simulink model "Modelo_PO"  (R2023b)
settings: Solver=ode23tb  StartTime=0.0  StopTime=60  RelTol=1e-4
values from neighbouring files (symbols this model uses):
  selector = i    [AA_Simulacion.m]
undefined symbols (not defined in the file or in its folder): sigbuilder_block
libraries: simulink x5, spsSeriesRLCBranchLib x4, spsDiodeLib x2, spsCurrentMeasurementLib x1, spsIGBTLib x1, spsPWMGeneratorDCDCLib x1, spsPVArrayLib x1, spsVoltageMeasurementLib x1, spspowerguiLib x1
settings Model: Creator=Guillermo  LastModifiedBy=Guillermo
settings DebuggingCC: MaskedZcDiagnostic=none  IgnoredZcDiagnostic=none  UnconnectedInputMsg=warning  UnconnectedOutputMsg=warning  UnconnectedLineMsg=warning
settings ModelReferenceCC: EnableRefExpFcnMdlSchedulingChecks=on
settings RTWCC: DLArmComputeVersion=19.05

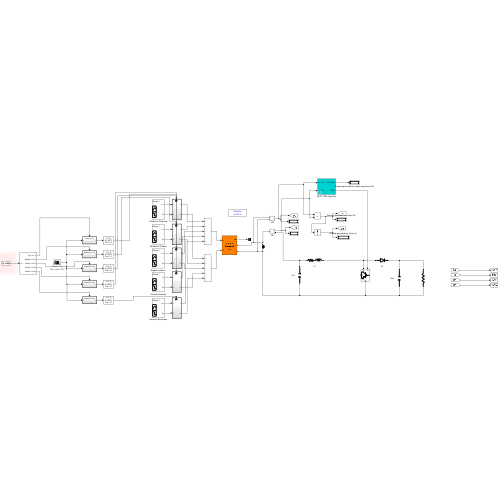
[thumbnail: Simulink's stored preview of the top-level diagram]
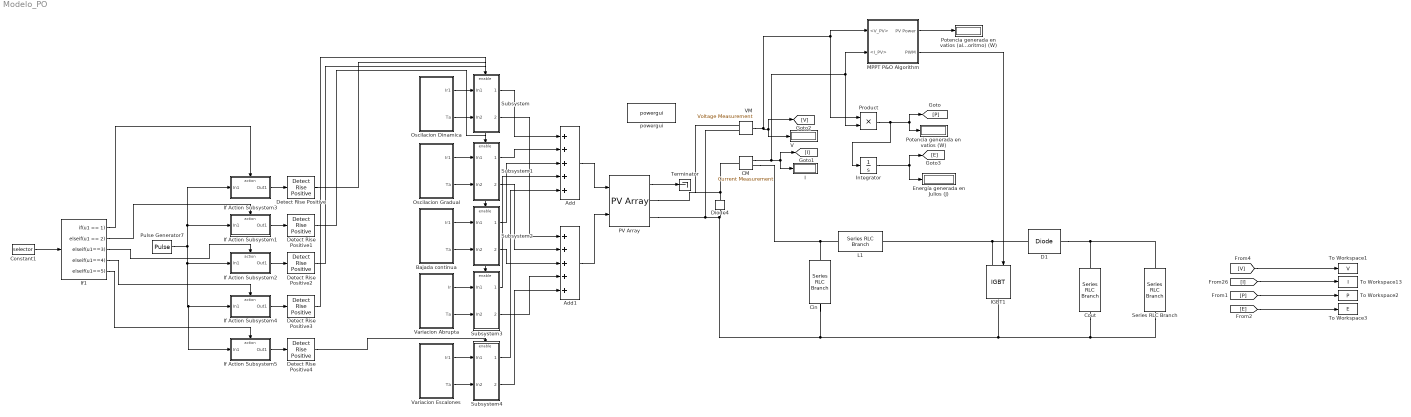
== system Modelo_PO ==
  Add : Sum  Inputs=+++++
  Add1 : Sum  Inputs=+++++
  Bajada continua : Subsystem  Tag=STV Subsys  LoadFcn=sigbuilder_block('load');  StartFcn=sigbuilder_block('start');  StopFcn=sigbuilder_block('stop');  ClipboardFcn=sigbuilder_block('clipboard');  mask(Sigbuilder block){tuvar=[0:10]}
      mask help: Simulink:masks:SigbuilderBlock_MD
      mask init:
      | if ~strcmp(get_param(bdroot(gcbh),'SimulationStatus'),'stopped') tuvar = sigbuilder_block('maskInit'); end
      settings: CopyFcn=sigbuilder_block('copy');  DeleteFcn=sigbuilder_block('delete');  ModelCloseFcn=sigbuilder_block('modelClose');  PreSaveFcn=sigbuilder_block('preSave');  PauseFcn=sigbuilder_block('pause');  ContinueFcn=sigbuilder_block('continue');  NameChangeFcn=sigbuilder_block('namechange');  OpenFcn=sigbuilder_block('open',[6 6 1012.5 506.25 ]);  CloseFcn=sigbuilder_block('close');
      mask Display: plot(0, 0, 100, 100,[2, 2, 32, 32, 2], [68, 8, 8, 68, 68],[32, 2], [38, 38], [32, 19, 2],[53, 60, 44], [32, 17, 17, 2],[16, 16, 31, 31]);txt = getActiveGroup(gcbh);text(2, 100, txt,'verticalAlignment', 'top');
  CM : spsCurrentMeasurementLib/Current Measurement  PhasorSimulation=off  OutputType=Complex  PSBequivalent=0
  Cin : spsSeriesRLCBranchLib/Series RLC Branch  LConnTagsString=__new0  RConnTagsString=__new0  BranchType=C  Resistance=0  Inductance=0  SetiL0=off  InitialCurrent=0  Capacitance=100e-6  Setx0=off  InitialVoltage=0  Measurements=None
  Constant1 : Constant  Value=selector
  Cout : spsSeriesRLCBranchLib/Series RLC Branch  LConnTagsString=__new0  RConnTagsString=__new0  BranchType=C  Resistance=0  Inductance=0  SetiL0=off  InitialCurrent=0  Capacitance=12000e-6  Setx0=off  InitialVoltage=0  Measurements=None
  D1 : spsDiodeLib/Diode  Ron=0.001  Lon=0  Vf=0.8  IC=0  UseSnubber=off  Rs=inf  Cs=250e-9  Measurements=off
  Detect Rise Positive{,1..4} (5 alike) : simulink/Logic and Bit Operations/Detect Rise Positive  vinit=0  OutDataTypeStr=boolean
  Diode4 : spsDiodeLib/Diode  Ron=0.001  Lon=0  Vf=0.7  IC=0  UseSnubber=0  Rs=500  Cs=250e-9  Measurements=off
  "Energía generada en Julios (J) " : Display
  I : Display
  IGBT1 : spsIGBTLib/IGBT  Ron=0.001  Lon=0  Vf=1  Tf=1e-6  Tt=2e-6  IC=0  Rs=1e5  Cs=inf  Measurements=off
  If Action Subsystem1 : Subsystem  TreatAsAtomicUnit=on
  If Action Subsystem2 : Subsystem  TreatAsAtomicUnit=on
  If Action Subsystem3 : Subsystem  TreatAsAtomicUnit=on
  If Action Subsystem4 : Subsystem  TreatAsAtomicUnit=on
  If Action Subsystem5 : Subsystem  TreatAsAtomicUnit=on
  If1 : If  IfExpression=u1 == 1  ElseIfExpressions=u1 == 2, u1==3, u1==4, u1==5  ShowElse=off
  Integrator : Integrator  ZeroCross=off
  L1 : spsSeriesRLCBranchLib/Series RLC Branch  LConnTagsString=__new0  RConnTagsString=__new0  BranchType=RL  Resistance=0  Inductance=0.005  SetiL0=off  InitialCurrent=0  Capacitance=100e-6  Setx0=off  InitialVoltage=0  Measurements=None
  MPPT P&O Algorithm : Subsystem  mask(MPPT Perturb and Observe Algorithm Block){Fsw=1000, StepSize=1e-6}
      mask prompts: Fsw "PWM Switching frequency (Hz):"; StepSize "PWM Duty Cycle (delta) Step Size"
      mask help:
      | MPPT Perturb & Observe Algorithm Block
      | Developed by Rodney Tan (PhD)
      | Version 1.00 Sep 2019
      |
      | This block perform photovoltaic panel Maximum Power Point Tracking based on Perturb & Observe algorithm.
      | This MPPT P&O method is implemented using basic Simulink block only.
      | This MPPT block take in Voltage and Current from photovoltaic panel and output PWM switching signal to drive the DC converter
      mask Help:
      | <b><u>Block Setting</u></b>
      | <b>PWM Switching Frequency (Hz)</b>
      | Specify the PWM switching frequency in Hz.
      | 
      | <b>PWM Duty Cycle Step Size</b>
      | Specify the PWM duty cycle (delta) step size. Default value is 1e-6.
      mask TypeOptions Fsw:
      | PWM Generator
      | (DC-DC)/Fsw
  Oscilacion Dinamica : Subsystem  Tag=STV Subsys  LoadFcn=sigbuilder_block('load');  StartFcn=sigbuilder_block('start');  StopFcn=sigbuilder_block('stop');  ClipboardFcn=sigbuilder_block('clipboard');  mask(Sigbuilder block){tuvar=[0:10]}
      mask help: Simulink:masks:SigbuilderBlock_MD
      mask init:
      | if ~strcmp(get_param(bdroot(gcbh),'SimulationStatus'),'stopped') tuvar = sigbuilder_block('maskInit'); end
      settings: CopyFcn=sigbuilder_block('copy');  DeleteFcn=sigbuilder_block('delete');  ModelCloseFcn=sigbuilder_block('modelClose');  PreSaveFcn=sigbuilder_block('preSave');  PauseFcn=sigbuilder_block('pause');  ContinueFcn=sigbuilder_block('continue');  NameChangeFcn=sigbuilder_block('namechange');  OpenFcn=sigbuilder_block('open',[12.75 -266.25 1012.5 506.25 ]);  CloseFcn=sigbuilder_block('close');
      mask Display: plot(0, 0, 100, 100,[2, 2, 32, 32, 2], [68, 8, 8, 68, 68],[32, 2], [38, 38], [32, 19, 2],[53, 60, 44], [32, 17, 17, 2],[16, 16, 31, 31]);txt = getActiveGroup(gcbh);text(2, 100, txt,'verticalAlignment', 'top');
  Oscilacion Gradual : Subsystem  Tag=STV Subsys  LoadFcn=sigbuilder_block('load');  StartFcn=sigbuilder_block('start');  StopFcn=sigbuilder_block('stop');  ClipboardFcn=sigbuilder_block('clipboard');  mask(Sigbuilder block){tuvar=[0:10]}
      mask help: Simulink:masks:SigbuilderBlock_MD
      mask init:
      | if ~strcmp(get_param(bdroot(gcbh),'SimulationStatus'),'stopped') tuvar = sigbuilder_block('maskInit'); end
      settings: CopyFcn=sigbuilder_block('copy');  DeleteFcn=sigbuilder_block('delete');  ModelCloseFcn=sigbuilder_block('modelClose');  PreSaveFcn=sigbuilder_block('preSave');  PauseFcn=sigbuilder_block('pause');  ContinueFcn=sigbuilder_block('continue');  NameChangeFcn=sigbuilder_block('namechange');  OpenFcn=sigbuilder_block('open',[4.5 30.75 1019.25 481.5 ]);  CloseFcn=sigbuilder_block('close');
      mask Display: plot(0, 0, 100, 100,[2, 2, 32, 32, 2], [68, 8, 8, 68, 68],[32, 2], [38, 38], [32, 19, 2],[53, 60, 44], [32, 17, 17, 2],[16, 16, 31, 31]);txt = getActiveGroup(gcbh);text(2, 100, txt,'verticalAlignment', 'top');
  PV Array : spsPVArrayLib/PV Array  Npar=1  Nser=1  PlotType=array @ 1000 W/m2 & specified temperatures  S_vec="[ 1000  500  100 ]"  Temp_C_vec="[ 45 25  ]"  ModuleName=SunPower SPR-305E-WHT-D  PlotWhenSelected=off  Pm=305.226  Ncell=96  Voc=64.2  Isc=5.96  Vm=54.7  Im=5.58  beta_Voc_pc=-0.2727  alpha_Isc_pc=0.061745  beta_Voc=-0.17507  alpha_Isc=0.00368  IL=5.9657  I0=6.3076e-12  nI=0.94489  Rsh=393.2054  Rs=0.37428  RobustModel=off  RobustCellTemperature=22.6  BAL=on  Tc=1e-3  Tfilter=5e-5
  "Potencia generada en vatios (W) " : Display
  Potencia generada en vatios (algoritmo) (W) : Display
  Product : Product
  Pulse Generator7 : DiscretePulseGenerator  PulseType=Time based  Period=1e-3  PulseWidth=20
      settings: AttributesFormatString=Period: %<period>\nDuty cycle: %<pulsewidth>%
  Series RLC Branch : spsSeriesRLCBranchLib/Series RLC Branch  LConnTagsString=__new0  RConnTagsString=__new0  BranchType=R  Resistance=500  Inductance=1e-3  SetiL0=off  InitialCurrent=0  Capacitance=1e-6  Setx0=off  InitialVoltage=0  Measurements=None
  Subsystem : Subsystem
  Subsystem1 : Subsystem
  Subsystem2 : Subsystem
  Subsystem3 : Subsystem
  Subsystem4 : Subsystem
  Terminator : Terminator
  To Workspace1 : ToWorkspace  VariableName=V  SampleTime=1e-3
  To Workspace13 : ToWorkspace  VariableName=I  SampleTime=1e-3
  To Workspace2 : ToWorkspace  VariableName=P  SampleTime=1e-3
  To Workspace3 : ToWorkspace  VariableName=E  SampleTime=1e-3
  V : Display
  VM : spsVoltageMeasurementLib/Voltage Measurement  PhasorSimulation=off  OutputType=Complex  PSBequivalent=0
  Variacion Abrupta : Subsystem  Tag=STV Subsys  LoadFcn=sigbuilder_block('load');  StartFcn=sigbuilder_block('start');  StopFcn=sigbuilder_block('stop');  ClipboardFcn=sigbuilder_block('clipboard');  mask(Sigbuilder block){tuvar=[0:10]}
      mask help: Simulink:masks:SigbuilderBlock_MD
      mask init:
      | if ~strcmp(get_param(bdroot(gcbh),'SimulationStatus'),'stopped') tuvar = sigbuilder_block('maskInit'); end
      settings: CopyFcn=sigbuilder_block('copy');  DeleteFcn=sigbuilder_block('delete');  ModelCloseFcn=sigbuilder_block('modelClose');  PreSaveFcn=sigbuilder_block('preSave');  PauseFcn=sigbuilder_block('pause');  ContinueFcn=sigbuilder_block('continue');  NameChangeFcn=sigbuilder_block('namechange');  OpenFcn=sigbuilder_block('open',[6 6 1012.5 506.25 ]);  CloseFcn=sigbuilder_block('close');
      mask Display: plot(0, 0, 100, 100,[2, 2, 32, 32, 2], [68, 8, 8, 68, 68],[32, 2], [38, 38], [32, 19, 2],[53, 60, 44], [32, 17, 17, 2],[16, 16, 31, 31]);txt = getActiveGroup(gcbh);text(2, 100, txt,'verticalAlignment', 'top');
  Variacion Escalones : Subsystem  Tag=STV Subsys  LoadFcn=sigbuilder_block('load');  StartFcn=sigbuilder_block('start');  StopFcn=sigbuilder_block('stop');  ClipboardFcn=sigbuilder_block('clipboard');  mask(Sigbuilder block){tuvar=[0:10]}
      mask help: Simulink:masks:SigbuilderBlock_MD
      mask init:
      | if ~strcmp(get_param(bdroot(gcbh),'SimulationStatus'),'stopped') tuvar = sigbuilder_block('maskInit'); end
      settings: CopyFcn=sigbuilder_block('copy');  DeleteFcn=sigbuilder_block('delete');  ModelCloseFcn=sigbuilder_block('modelClose');  PreSaveFcn=sigbuilder_block('preSave');  PauseFcn=sigbuilder_block('pause');  ContinueFcn=sigbuilder_block('continue');  NameChangeFcn=sigbuilder_block('namechange');  OpenFcn=sigbuilder_block('open',[6 6 1012.5 506.25 ]);  CloseFcn=sigbuilder_block('close');
      mask Display: plot(0, 0, 100, 100,[2, 2, 32, 32, 2], [68, 8, 8, 68, 68],[32, 2], [38, 38], [32, 19, 2],[53, 60, 44], [32, 17, 17, 2],[16, 16, 31, 31]);txt = getActiveGroup(gcbh);text(2, 100, txt,'verticalAlignment', 'top');
  powergui : spspowerguiLib/powergui  Priority=1  SimulationMode=Discrete  SampleTime=1e-5  frequency=60  Iterations=50  frequencyindice=0  Pbase=100e6  ErrMax=1e-4  UnitsV=kV  UnitsW=MW  buscounter=0  FunctionMessages=off  echomessages=off  EnableUseOfTLC=off  CurrentSourceSwitches=on  DisableSnubberDevices=on  DisableRonSwitches=off  DisableVfSwitches=off  DisplayEquations=off  AutomaticDiscreteSolvers=off  SolverType=Tustin/Backward Euler (TBE)  Interpol=off  ExternalGateDelay=off  methode=off  Ts=0  x0status=blocks  SPID=off  SwTol=0  HookPort=off  NonlinearTolerance=1e-4  nMaxIteration=100  ContinueOnMaxIteration=off  RestoreLinks=warning  ResistiveCurrentMeasurement=off  Frange=[0:2:500]  Ylog=off  Xlog=on  ShowGrid=off  save=off  variable=ZData  structure=0  ZoomFFT=on  StartTime=0.0  cycles=1  DisplayStyle=1  fundamental=60  FreqAxis=off  MaxFrequency=1000  frequencyindicesteady=1  RmsSteady=1  display=off
  wires:
  [V] -> To Workspace1/1
  VM/1 -> Product/1, MPPT P&O Algorithm/1(<V_PV>), [V], V/1
  CM/1 -> I/1, [I], Product/2, MPPT P&O Algorithm/2(<I_PV>)
  PV Array/1 -> Terminator/1
  [I] -> To Workspace13/1
  Integrator/1 -> [E], "Energía generada en Julios (J) "/1
  [P] -> To Workspace2/1
  [E] -> To Workspace3/1
  MPPT P&O Algorithm/2(PWM) -> IGBT1/1
  MPPT P&O Algorithm/1(PV Power) -> Potencia generada en vatios (algoritmo) (W)/1
  Product/1 -> Integrator/1, "Potencia generada en vatios (W) "/1, [P]
  Subsystem2/1(Out1) -> Add/3
  Subsystem/2(Out2) -> Add1/1
  Subsystem4/1(Out1) -> Add/5
  If Action Subsystem1/1(Out1) -> Detect Rise Positive1/1
  Oscilacion Gradual/1(Ir1) -> Subsystem1/1(In1)
  Oscilacion Dinamica/2(Ta) -> Subsystem/2(In2)
  If Action Subsystem5/1(Out1) -> Detect Rise Positive4/1
  Subsystem/1(Out1) -> Add/1
  Subsystem1/2(Out2) -> Add1/2
  Subsystem2/2(Out2) -> Add1/3
  Subsystem3/2(Out2) -> Add1/4
  Variacion Abrupta/2(Ta) -> Subsystem3/2(In2)
  Oscilacion Dinamica/1(Ir1) -> Subsystem/1(In1)
  If1/1 -> If Action Subsystem3/Action
  Variacion Escalones/2(Ta) -> Subsystem4/2(In2)
  Detect Rise Positive/1 -> Subsystem/Enable
  If1/5 -> If Action Subsystem5/Action
  If Action Subsystem4/1(Out1) -> Detect Rise Positive3/1
  Subsystem4/2(Out2) -> Add1/5
  Variacion Abrupta/1(Ir) -> Subsystem3/1(In1)
  Subsystem3/1(Out1) -> Add/4
  Bajada continua/1(Ir1) -> Subsystem2/1(In1)
  If1/3 -> If Action Subsystem2/Action
  Constant1/1 -> If1/1
  Pulse Generator7/1 -> If Action Subsystem3/1(In1), If Action Subsystem1/1(In1), If Action Subsystem5/1(In1), If Action Subsystem4/1(In1), If Action Subsystem2/1(In1)
  Subsystem1/1(Out1) -> Add/2
  Bajada continua/2(Ta) -> Subsystem2/2(In2)
  If Action Subsystem2/1(Out1) -> Detect Rise Positive2/1
  If1/2 -> If Action Subsystem1/Action
  If1/4 -> If Action Subsystem4/Action
  Variacion Escalones/1(Ir1) -> Subsystem4/1(In1)
  If Action Subsystem3/1(Out1) -> Detect Rise Positive/1
  Oscilacion Gradual/2(Ta) -> Subsystem1/2(In2)
  Add/1 -> PV Array/1
  Add1/1 -> PV Array/2
  Detect Rise Positive1/1 -> Subsystem1/Enable
  Detect Rise Positive2/1 -> Subsystem2/Enable
  Detect Rise Positive3/1 -> Subsystem3/Enable
  Detect Rise Positive4/1 -> Subsystem4/Enable
  connections:
  D1/LConn1 -- IGBT1/LConn1 -- L1/RConn1
  PV Array/RConn2 -- VM/LConn2 -- Cin/RConn1 -- Cout/RConn1 -- Series RLC Branch/RConn1 -- IGBT1/RConn1 -- Diode4/LConn1
  Series RLC Branch/LConn1 -- D1/RConn1 -- Cout/LConn1
  Diode4/RConn1 -- VM/LConn1 -- PV Array/RConn1 -- CM/LConn1
  CM/RConn1 -- Cin/LConn1 -- L1/LConn1

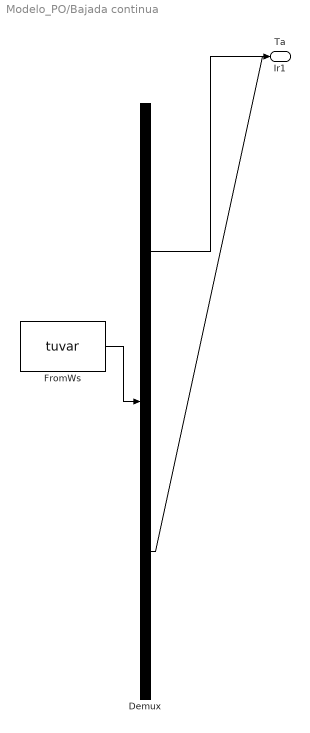
== system Modelo_PO/Bajada continua ==
  Demux : Demux  Tag=STV Demux  Outputs=2
      settings: DisplayOption=none
  FromWs : FromWorkspace  Tag=STV FromWs  VariableName=tuvar
      SigBuilderData=|
      | common.afterFinalStr = 'Extrapolate'
      | common.sampleTime = 0
      | dataSet.timeRange = [0 60]
      | dataSet.name = 'Group 1'
      | sbobj.Groups.Name = 'Group 1'
      | sbobj.Groups.Signals(1).Name = 'Ir1'
      | sbobj.Groups.Signals(1).XData = [0 60]
      | sbobj.Groups.Signals(1).YData = [1000 0]
      | sbobj.Groups.Signals(2).Name = 'Ta'
      | sbobj.Groups.Signals(2).XData = [0 60]
      | sbobj.Groups.Signals(2).YData = [22.6 22.6]
      | sbobj.Groups.TimeRange = [0 60]
  Ir1 : Outport  Tag=STV Outport
  Ta : Outport  Tag=STV Outport  Port=2
  wires:
  FromWs/1 -> Demux/1
  Demux/1 -> Ir1/1
  Demux/2 -> Ta/1

== system Modelo_PO/If Action Subsystem1 ==
  In1 : Inport
  Action Port : ActionPort  InitializeStates=reset  ActionPortLabel=elseif(u1 == 2)
  Out1 : Outport
  wires:
  In1/1 -> Out1/1

== system Modelo_PO/If Action Subsystem2 ==
  In1 : Inport
  Action Port : ActionPort  InitializeStates=reset  ActionPortLabel=elseif( u1==3)
  Out1 : Outport
  wires:
  In1/1 -> Out1/1

== system Modelo_PO/If Action Subsystem3 ==
  In1 : Inport
  Action Port : ActionPort  InitializeStates=reset  ActionPortLabel=if(u1 == 1)
  Out1 : Outport
  wires:
  In1/1 -> Out1/1

== system Modelo_PO/If Action Subsystem4 ==
  In1 : Inport
  Action Port : ActionPort  InitializeStates=reset  ActionPortLabel=elseif( u1==4)
  Out1 : Outport
  wires:
  In1/1 -> Out1/1

== system Modelo_PO/If Action Subsystem5 ==
  In1 : Inport
  Action Port : ActionPort  InitializeStates=reset  ActionPortLabel=elseif( u1==5)
  Out1 : Outport
  wires:
  In1/1 -> Out1/1

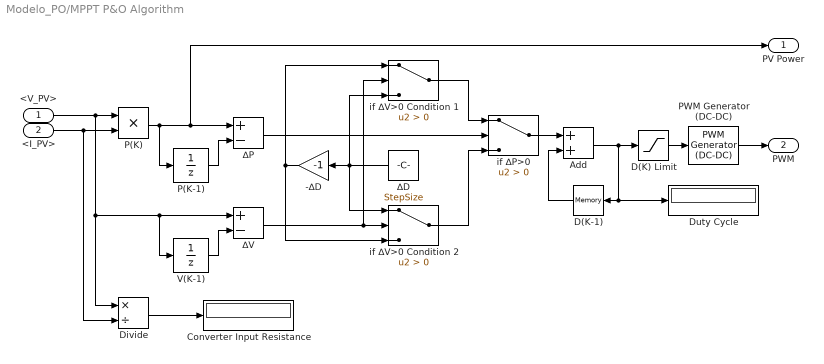
== system Modelo_PO/MPPT P&O Algorithm ==
  <V_PV> : Inport
  <I_PV> : Inport  Port=2
  -∆D : Gain  Gain=-1
  Add : Sum
  Converter Input Resistance : Display
  D(K) Limit : Saturate  UpperLimit=1  LowerLimit=0
  D(K-1) : Memory  InitialCondition=0.5  InheritSampleTime=on
  Divide : Product  Inputs=*/
  Duty Cycle : Display
  P(K) : Product
  P(K-1) : UnitDelay  SampleTime=-1  HasFrameUpgradeWarning=on
  PWM Generator (DC-DC) : spsPWMGeneratorDCDCLib/PWM Generator (DC-DC)  Fsw=Fsw  Ts=0
  V(K-1) : UnitDelay  SampleTime=-1  HasFrameUpgradeWarning=on
  if ∆P>0 : Switch  Criteria=u2 > Threshold  SaturateOnIntegerOverflow=off  InputSameDT=off
  if ∆V>0 Condition 1 : Switch  Criteria=u2 > Threshold  SaturateOnIntegerOverflow=off  InputSameDT=off
  if ∆V>0 Condition 2 : Switch  Criteria=u2 > Threshold  SaturateOnIntegerOverflow=off  InputSameDT=off
  ∆D : Constant  Value=StepSize
  ∆P : Sum  Inputs=+-
  ∆V : Sum  Inputs=+-
  PV Power : Outport  VectorParamsAs1DForOutWhenUnconnected=off
  PWM : Outport  Port=2  VectorParamsAs1DForOutWhenUnconnected=off
  wires:
  P(K)/1 -> ∆P/1, PV Power/1, P(K-1)/1
  <I_PV>/1 -> P(K)/2, Divide/2
  if ∆P>0/1 -> Add/1
  if ∆V>0 Condition 1/1 -> if ∆P>0/1
  ∆P/1 -> if ∆P>0/2
  P(K-1)/1 -> ∆P/2
  V(K-1)/1 -> ∆V/2
  ∆V/1 -> if ∆V>0 Condition 2/2, if ∆V>0 Condition 1/2
  <V_PV>/1 -> Divide/1, ∆V/1, V(K-1)/1, P(K)/1
  Add/1 -> D(K) Limit/1, Duty Cycle/1, D(K-1)/1
  if ∆V>0 Condition 2/1 -> if ∆P>0/3
  D(K-1)/1 -> Add/2
  ∆D/1 -> if ∆V>0 Condition 2/1, -∆D/1, if ∆V>0 Condition 1/3
  -∆D/1 -> if ∆V>0 Condition 2/3, if ∆V>0 Condition 1/1
  PWM Generator (DC-DC)/1 -> PWM/1
  Divide/1 -> Converter Input Resistance/1
  D(K) Limit/1 -> PWM Generator (DC-DC)/1

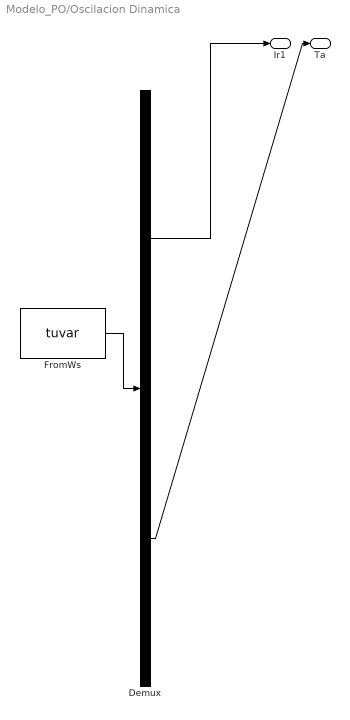
== system Modelo_PO/Oscilacion Dinamica ==
  Demux : Demux  Tag=STV Demux  Outputs=2
      settings: DisplayOption=none
  FromWs : FromWorkspace  Tag=STV FromWs  VariableName=tuvar
      SigBuilderData=|
      | common.afterFinalStr = 'Extrapolate'
      | common.sampleTime = 0
      | dataSet.timeRange = [0 60]
      | dataSet.name = 'Group 1'
      | sbobj.Groups.Name = 'Group 1'
      | sbobj.Groups.Signals(1).Name = 'Ir1'
      | sbobj.Groups.Signals(1).XData = [0 1 1.4 7 7.25 10 10.25 10.5 12 12.25 16 16.25 16.5 16.75 18.95 19.5 20 21.05 24 24.5 25 25.25 25.75 29 32 32.25 34 34.25 34.5 34.75 35 37 37.25 41 41.25 41.5 41.75 42 45 45.25 48 48.25 50 50.25 53.75 54 54.25 57 57.25 60]
      | sbobj.Groups.Signals(1).YData = [910 500 295 295 910 910 295 295 295 910 910 295 910 295 295 910 295 910 910 290 910 295 910 910 910 295 295 910 295 910 295 295 910 910 295 910 295 910 910 295 295 910 910 295 295 910 295 295 790 790]
      | sbobj.Groups.Signals(2).Name = 'Ta'
      | sbobj.Groups.Signals(2).XData = [0 60]
      | sbobj.Groups.Signals(2).YData = [22.6 22.6]
      | sbobj.Groups.TimeRange = [0 60]
  Ir1 : Outport  Tag=STV Outport
  Ta : Outport  Tag=STV Outport  Port=2
  wires:
  FromWs/1 -> Demux/1
  Demux/1 -> Ir1/1
  Demux/2 -> Ta/1

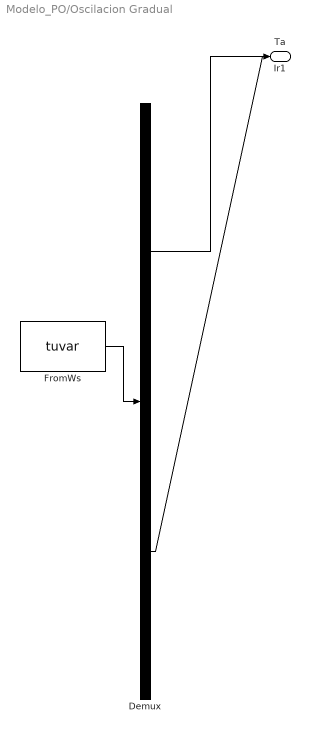
== system Modelo_PO/Oscilacion Gradual ==
  Demux : Demux  Tag=STV Demux  Outputs=2
      settings: DisplayOption=none
  FromWs : FromWorkspace  Tag=STV FromWs  VariableName=tuvar
      SigBuilderData=|
      | common.afterFinalStr = 'Extrapolate'
      | common.sampleTime = 0
      | dataSet.timeRange = [0 60]
      | dataSet.name = 'Group 1'
      | sbobj.Groups.Name = 'Group 1'
      | sbobj.Groups.Signals(1).Name = 'Ir1'
      | sbobj.Groups.Signals(1).XData = [0 1 1.4 7 7.25 16.5 16.75 25.25 25.75 34.75 35 37 37.25 45 45.25 48 48.25 50 50.25 57 57.25 57.25 60]
      | sbobj.Groups.Signals(1).YData = [910 500 295 295 910 910 295 295 910 910 295 295 910 910 295 295 910 910 295 295 775 800 800]
      | sbobj.Groups.Signals(2).Name = 'Ta'
      | sbobj.Groups.Signals(2).XData = [0 60]
      | sbobj.Groups.Signals(2).YData = [22.6 22.6]
      | sbobj.Groups.TimeRange = [0 60]
  Ir1 : Outport  Tag=STV Outport
  Ta : Outport  Tag=STV Outport  Port=2
  wires:
  FromWs/1 -> Demux/1
  Demux/1 -> Ir1/1
  Demux/2 -> Ta/1

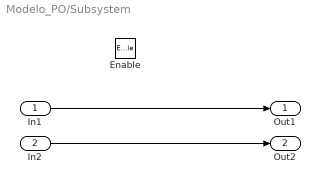
== system Modelo_PO/Subsystem ==
  In1 : Inport
  In2 : Inport  Port=2
  Enable : EnablePort
  Out1 : Outport
  Out2 : Outport  Port=2
  wires:
  In1/1 -> Out1/1
  In2/1 -> Out2/1

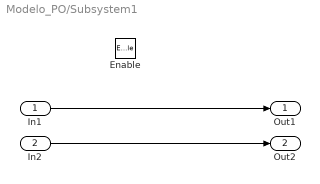
== system Modelo_PO/Subsystem1 ==
  In1 : Inport
  In2 : Inport  Port=2
  Enable : EnablePort
  Out1 : Outport
  Out2 : Outport  Port=2
  wires:
  In1/1 -> Out1/1
  In2/1 -> Out2/1

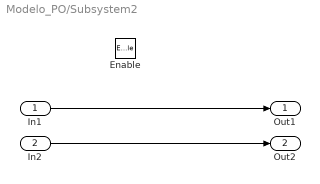
== system Modelo_PO/Subsystem2 ==
  In1 : Inport
  In2 : Inport  Port=2
  Enable : EnablePort
  Out1 : Outport
  Out2 : Outport  Port=2
  wires:
  In1/1 -> Out1/1
  In2/1 -> Out2/1

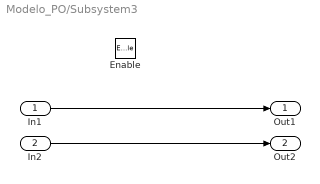
== system Modelo_PO/Subsystem3 ==
  In1 : Inport
  In2 : Inport  Port=2
  Enable : EnablePort
  Out1 : Outport
  Out2 : Outport  Port=2
  wires:
  In1/1 -> Out1/1
  In2/1 -> Out2/1

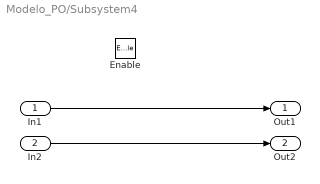
== system Modelo_PO/Subsystem4 ==
  In1 : Inport
  In2 : Inport  Port=2
  Enable : EnablePort
  Out1 : Outport
  Out2 : Outport  Port=2
  wires:
  In1/1 -> Out1/1
  In2/1 -> Out2/1

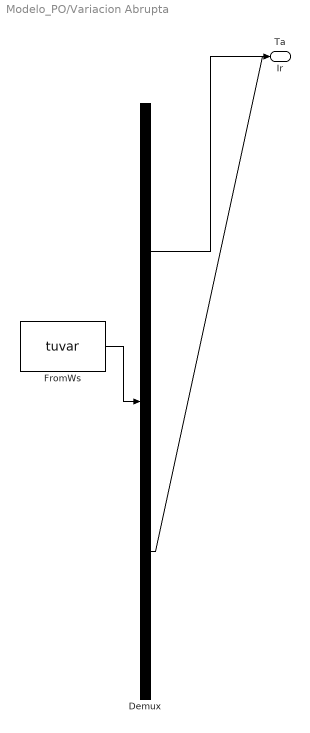
== system Modelo_PO/Variacion Abrupta ==
  Demux : Demux  Tag=STV Demux  Outputs=2
      settings: DisplayOption=none
  FromWs : FromWorkspace  Tag=STV FromWs  VariableName=tuvar
      SigBuilderData=|
      | common.afterFinalStr = 'Extrapolate'
      | common.sampleTime = 0
      | dataSet.timeRange = [0 60]
      | dataSet.name = 'Group 1'
      | sbobj.Groups.Name = 'Group 1'
      | sbobj.Groups.Signals(1).Name = 'Ir'
      | sbobj.Groups.Signals(1).XData = [0 20 20.1 40 40.1 60]
      | sbobj.Groups.Signals(1).YData = [800 800 100 100 600 600]
      | sbobj.Groups.Signals(2).Name = 'Ta'
      | sbobj.Groups.Signals(2).XData = [0 60]
      | sbobj.Groups.Signals(2).YData = [22.6 22.6]
      | sbobj.Groups.TimeRange = [0 60]
  Ir : Outport  Tag=STV Outport
  Ta : Outport  Tag=STV Outport  Port=2
  wires:
  FromWs/1 -> Demux/1
  Demux/1 -> Ir/1
  Demux/2 -> Ta/1

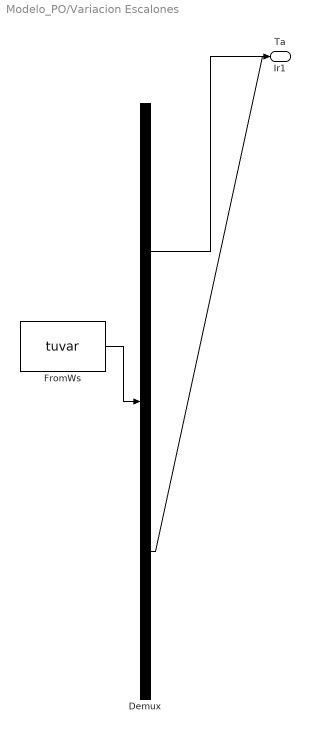
== system Modelo_PO/Variacion Escalones ==
  Demux : Demux  Tag=STV Demux  Outputs=2
      settings: DisplayOption=none
  FromWs : FromWorkspace  Tag=STV FromWs  VariableName=tuvar
      SigBuilderData=|
      | common.afterFinalStr = 'Extrapolate'
      | common.sampleTime = 0
      | dataSet.timeRange = [0 60]
      | dataSet.name = 'Group 1'
      | sbobj.Groups.Name = 'Group 1'
      | sbobj.Groups.Signals(1).Name = 'Ir1'
      | sbobj.Groups.Signals(1).XData = [0 15 15.1 30 30.1 45 45.1 60]
      | sbobj.Groups.Signals(1).YData = [1200 1200 900 900 600 600 300 300]
      | sbobj.Groups.Signals(2).Name = 'Ta'
      | sbobj.Groups.Signals(2).XData = [0 60]
      | sbobj.Groups.Signals(2).YData = [22.6 22.6]
      | sbobj.Groups.TimeRange = [0 60]
  Ir1 : Outport  Tag=STV Outport
  Ta : Outport  Tag=STV Outport  Port=2
  wires:
  FromWs/1 -> Demux/1
  Demux/1 -> Ir1/1
  Demux/2 -> Ta/1
